simulink model "estimador"  (R2021a)
settings: Solver=VariableStepAuto  StartTime=0.0  StopTime=10.0  RelTol=1e-3
values from neighbouring files (symbols this model uses):
  A1 = A-B*K-L*C    [Exe1-old.m]    (also in Exe1.m)
  B1 = L    [Exe1-old.m]    (also in Exe1.m)
  C1 = -K    [Exe1-old.m]    (also in Exe1.m)
  x0 = [0.1 0 0 0 0]'    [Exe1-old.m]    (also in Exe1.m)
undefined symbols (not defined in the file or in its folder): A, B, C, D
settings Model: Creator=Tiago  LastModifiedBy=Tiago

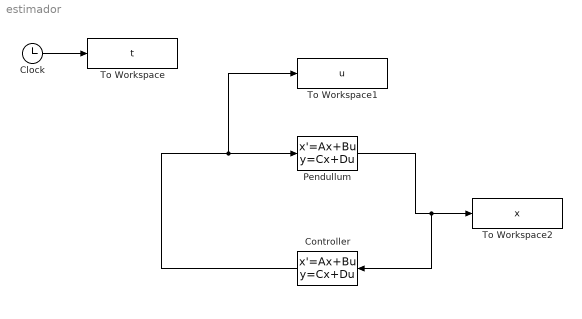
== system estimador ==
  Clock : Clock
  Controller : StateSpace  A=A1  B=B1  C=C1  D=D  InitialCondition=0
  Pendullum : StateSpace  A=A  B=B  C=C  D=D  InitialCondition=x0
  To Workspace : ToWorkspace  VariableName=t  SaveFormat=Timeseries  SampleTime=-1
  To Workspace1 : ToWorkspace  VariableName=u  SaveFormat=Timeseries  SampleTime=-1
  To Workspace2 : ToWorkspace  VariableName=x  SaveFormat=Timeseries  SampleTime=-1
  wires:
  Pendullum/1 -> Controller/1, To Workspace2/1
  Clock/1 -> To Workspace/1
  Controller/1 -> To Workspace1/1, Pendullum/1
